simulink model "pah"  (Simulink 10.0)
settings: Solver=ode15s  StartTime=0.0  StopTime=60  MaxStep=5  RelTol=1e-6  AbsTol=1e-6
undefined symbols (not defined in the file): Aelv, Belv, Celv, Delv, Ki_1, Kq, Ktheta, uaero0, uprop0, xinco
libraries: fbuttons x1, fdclib10 x1
settings Model: Creator=bhisma  LastModifiedBy=bhisma  ExtModeTrigMode=oneshot  ExtModeArmWhenConnect=off
settings DataIOCC: SignalLoggingSaveFormat=ModelDataLogs  SaveOutput=off  SaveTime=off
settings OptimizationCC: BlockReduction=off  BooleanDataType=off  LifeSpan=auto
settings DebuggingCC: SaveWithParameterizedLinksMsg=none  SignalResolutionControl=TryResolveAllWithWarning  MultiTaskDSMMsg=warning  MultiTaskCondExecSysMsg=none  SFUnexpectedBacktrackingDiag=error  SFNoUnconditionalDefaultTransitionDiag=error  SFExecutionAtInitializationDiag=warning  ArithmeticOperatorsInVariantConditions=error
settings HardwareCC: ProdBitPerPointer=64  ProdBitPerSizeT=64  ProdBitPerPtrDiffT=64  ProdLargestAtomicFloat=Float  ProdIntDivRoundTo=Zero  ProdEndianess=LittleEndian  ProdWordSize=64  ProdHWDeviceType=Intel->x86-64 (Windows64)  TargetUnknown=on
settings SFSimCC: SimUseLocalCustomCode=on  CustomCodeUndefinedFunction=FilterOut
settings RTWCC: TemplateMakefile=grt_vc.tmf  RTWUseLocalCustomCode=on
settings CodeAppCC: StateflowObjectComments=off
settings GRTTargetCC: TargetLangStandard=C99 (ISO)
settings ConfigComp: CovMetricSettings=dwe  CovHtmlReporting=off  CovSaveCumulativeToWorkspaceVar=off  CovSaveSingleToWorkspaceVar=off

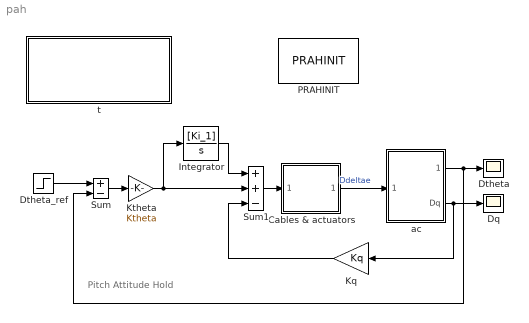
== system pah ==
  note: Pitch Attitude Hold
  Cables & actuators : Subsystem
      mask Display: disp('Cable &\nactuator\ndynamics')
  Dq : Scope
  Dtheta : Scope
  Dtheta_ref : Step  Time=0  After=1*pi/180  SampleTime=0
  Integrator : TransferFcn  Numerator=[Ki_1]  Denominator=[1 0]
  Kq : Gain  Gain=Kq  SaturateOnIntegerOverflow=on  OutDataTypeStr=Inherit: Same as input  ParamDataTypeStr=Inherit: Same as input
  Ktheta : Gain  Gain=Ktheta  SaturateOnIntegerOverflow=on  OutDataTypeStr=Inherit: Same as input  ParamDataTypeStr=Inherit: Same as input
  PRAHINIT : fbuttons/PRAHINIT
  Sum : Sum  Inputs=+-  SaturateOnIntegerOverflow=on  InputSameDT=on  OutDataTypeStr=Inherit: Same as first input
  Sum1 : Sum  Inputs=++-  SaturateOnIntegerOverflow=on  InputSameDT=on  OutDataTypeStr=Inherit: Same as first input
  ac : Subsystem
      mask Display: disp('BEAVER\ndynamics')
  t : Subsystem
      settings: OpenFcn=browse apilot
      mask Display: disp('Pitch Attitude Hold mode,\nwithout turn-compensation\n(no signal limiters).\nM.O. Rauw, May 2004')
  wires:
  ac/1(Dtheta) -> Sum/2, Dtheta/1
  ac/2(Dq) -> Kq/1, Dq/1
  Sum1/1 -> Cables & actuators/1(VDdeltae)
  Cables & actuators/1(Ddeltae) -> ac/1(Ddelta_e)  "Ddeltae"
  Sum/1 -> Ktheta/1
  Dtheta_ref/1 -> Sum/1
  Kq/1 -> Sum1/3
  Integrator/1 -> Sum1/1
  Ktheta/1 -> Integrator/1, Sum1/2

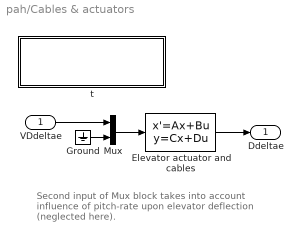
== system pah/Cables & actuators ==
  note: Second input of Mux block takes into account
      | influence of pitch-rate upon elevator deflection
      | (neglected here).
  VDdeltae : Inport
  Elevator actuator and cables : StateSpace  A=Aelv  B=Belv  C=Celv  D=Delv  InitialCondition=0
  Ground : Ground
  Mux : Mux  Inputs=2
  t : Subsystem
      settings: OpenFcn=browse actuatr
      mask Display: disp('Dynamics of the cables\nand actuator of the elevator\nM.O. Rauw, April 2003')
  Ddeltae : Outport
  wires:
  Elevator actuator and cables/1 -> Ddeltae/1
  Ground/1 -> Mux/2
  Mux/1 -> Elevator actuator and cables/1
  VDdeltae/1 -> Mux/1

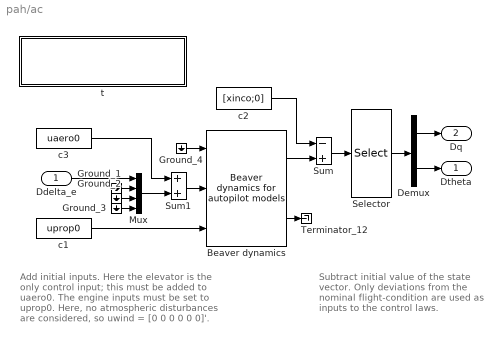
== system pah/ac ==
  note: Add initial inputs. Here the elevator
      | is the only control input; this must
      | be added to uaero0. The engine
      | inputs must be set to uprop0. Here,
      | no atmospheric disturbances are
      | considered, so uwind = [0 0 0 0 0 0]'.
  note: Subtract initial value of  the state
      | vector. Only deviations from the
      | nominal flight-condition are used
      | as inputs to the control laws.
  Ddelta_e : Inport
  Beaver dynamics : fdclib10/Beaver dynamics for autopilot models
  Demux : Demux  Outputs=2
  Ground_{1..4} (4 alike) : Ground
  Mux : Mux
  Selector : Selector  InputPortWidth=13  IndexOptions=Index vector (dialog)  Indices=[5 8]  OutputSizes=1
  Sum : Sum  Inputs=-+  SaturateOnIntegerOverflow=on  InputSameDT=on  OutDataTypeStr=Inherit: Same as first input
  Sum1 : Sum  SaturateOnIntegerOverflow=on  InputSameDT=on  OutDataTypeStr=Inherit: Same as first input
  Terminator_12 : Terminator
  c1 : Constant  Value=uprop0
  c2 : Constant  Value=[xinco;0]
  c3 : Constant  Value=uaero0
  t : Subsystem
      mask Display: disp('Call aircraft model and convert\nI/O signals to small-deviations.\nM.O. Rauw, January 2004')
  Dtheta : Outport
  Dq : Outport  Port=2
  wires:
  Sum/1 -> Selector/1
  Beaver dynamics/1 -> Sum/2
  c2/1 -> Sum/1
  Beaver dynamics/2 -> Terminator_12/1
  Ddelta_e/1 -> Mux/1
  Ground_3/1 -> Mux/4
  Ground_2/1 -> Mux/3
  Ground_1/1 -> Mux/2
  c3/1 -> Sum1/1
  Mux/1 -> Sum1/2
  Sum1/1 -> Beaver dynamics/2
  c1/1 -> Beaver dynamics/3
  Ground_4/1 -> Beaver dynamics/1
  Selector/1 -> Demux/1
  Demux/1 -> Dq/1
  Demux/2 -> Dtheta/1

== system pah/t ==

== system pah/Cables & actuators/t ==

== system pah/ac/t ==
